simulink model "Glucose_Iodine model"  (R2021a)
settings: Solver=VariableStepAuto  StartTime=0.0  StopTime=10.0  RelTol=1e-3
libraries: simulink x2
settings Model: Creator=SAT  LastModifiedBy=MSII

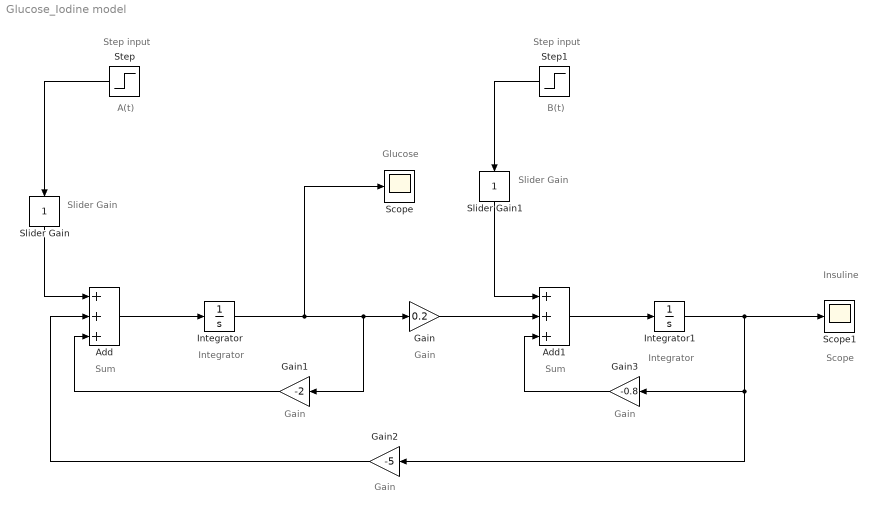
== system Glucose_Iodine model ==
  note: Gain
  note: Integrator
  note: Sum
  note: Insuline
  note: Glucose
  note: Slider
      | Gain
  note: Step input
  note: A(t)
  note: B(t)
  note: Step input
  note: Slider
      | Gain
  note: Scope
  note: Sum
  note: Integrator
  note: Gain
  note: Gain
  note: Gain
  Add : Sum  Inputs=+++
  Add1 : Sum  Inputs=+++
  Gain : Gain  Gain=0.2
  Gain1 : Gain  Gain=-2
  Gain2 : Gain  Gain=-5
  Gain3 : Gain  Gain=-0.8
  Integrator : Integrator
  Integrator1 : Integrator
  Scope : Scope
  Scope1 : Scope
  Slider Gain : simulink/Math Operations/Slider Gain  gain=1  low=0  high=2
  Slider Gain1 : simulink/Math Operations/Slider Gain  gain=1  low=0  high=2
  Step : Step  Before=1  SampleTime=0
  Step1 : Step  After=0  SampleTime=0
  wires:
  Step/1 -> Slider Gain/1
  Slider Gain/1 -> Add/1
  Add/1 -> Integrator/1
  Integrator/1 -> Scope/1, Gain1/1, Gain/1
  Gain/1 -> Add1/2
  Slider Gain1/1 -> Add1/1
  Step1/1 -> Slider Gain1/1
  Add1/1 -> Integrator1/1
  Integrator1/1 -> Gain3/1, Gain2/1, Scope1/1
  Gain1/1 -> Add/3
  Gain2/1 -> Add/2
  Gain3/1 -> Add1/3
